simulink model "ToySystem"  (R2019b)
settings: Solver=VariableStepAuto  StartTime=0.0  StopTime=10.0  RelTol=1e-3
undefined symbols (not defined in the file or in its folder): b1, b2, Cp_wall, D, dH, dH1, dH2, f, f1, f2, Fluid, Fluid1, Fluid2, H, HTC, HTC1, HTC2, HTC_method, HTC_method1, HTC_method2, KL, KL1, KL2, L, L1, L2, M_wall, Nu_lam1, Nu_lam2, P_init, PAF, Pamb, Pass1, Pass2, rev_comms_sink, Tw_init, v, W1, W2
libraries: DAEMOT_Lib x21
(part 2 of 2)

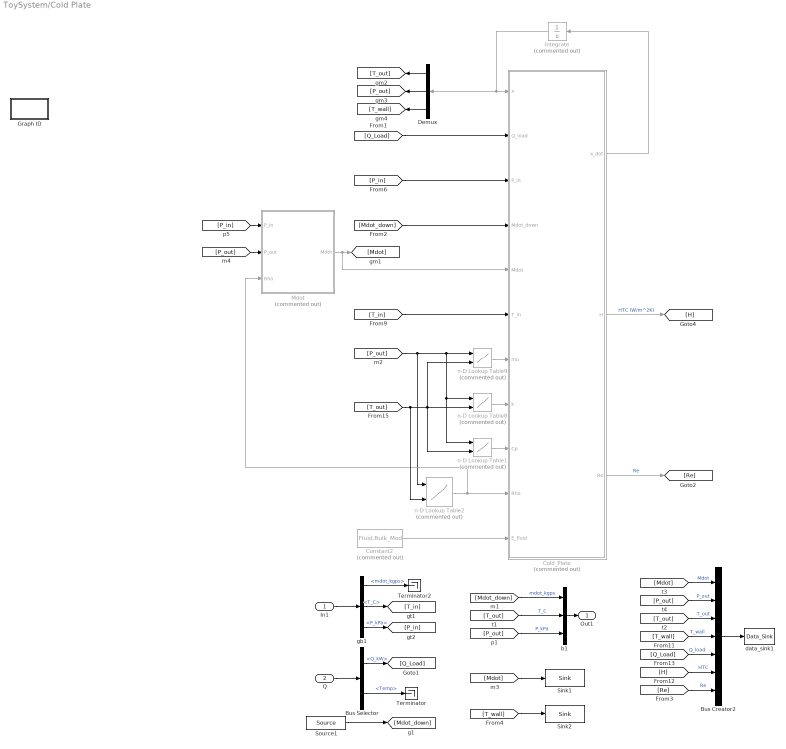
== system ToySystem/Cold Plate ==
  In1 : Inport
  Q : Inport  Port=2
  Bus Creator2 : BusCreator  Inputs=7
  Bus Selector : BusSelector  OutputSignals=Q_kW,Temp
  Cold_Plate : MATLAB Function  Commented=on  TreatAsAtomicUnit=on
  Constant2 : Constant  Commented=on  Value=Fluid.Bulk_Mod
  Demux : Demux  Outputs=3
  Graph ID : Subsystem  mask(Automated Graph Identifier){skip=off, graphType=HeatLoad, downCompType=SplitJunction, downCompPath=ToySystem/Junction, upCompType=Tank,Source, upCompPath=ToySystem/Tank 1,ToySystem/Generic Source1, spec=0}
      mask prompts: skip "Skip this block?"; graphType "Graph Type"; downCompType "Downstream Component Type"; downCompPath "Downstream Component Path"; upCompType "Upstream Component Type"; upCompPath "Upstream Component Path"; spec "Special"
      mask help: This block is used to generate directed graphs from DAEMOT models.
      mask init:
      | graph_connections()
      mask TypeOptions graphType: Tank | HeatExchanger | HeatLoad | SplitJunction | Source | Sink
      mask Callback graphType:
      | % grab the Simulink Mask object for this block
      | maskObj = Simulink.Mask.get(gcb);
      | 
      | % assign the popup with a list of graph options
      | maskObj.Parameters(2).TypeOptions = generateGraphList();
  Integrate : Integrator  Commented=on  InitialCondition=[T_init P_init Tw_init]
  Mdot : MATLAB Function  Commented=on  TreatAsAtomicUnit=on
  Sink1 : DAEMOT_Lib/Support Functions/Sink
      settings: SourceProductName=DAEMOT Toolset
  Sink2 : DAEMOT_Lib/Support Functions/Sink
      settings: SourceProductName=DAEMOT Toolset
  Source1 : DAEMOT_Lib/Support Functions/Source
      settings: SourceProductName=DAEMOT Toolset
  Terminator : Terminator
  Terminator2 : Terminator
  b1 : BusCreator  Inputs=3
  data_sink1 : DAEMOT_Lib/Support Functions/Data_Sink
      settings: SourceProductName=DAEMOT Toolset
  gb1 : BusSelector  OutputSignals=mdot_kgps,T_C,P_kPa
  n-D Lookup Table1 : Lookup_n-D  Commented=on  BreakpointsForDimension1=Fluid.P  BreakpointsForDimension2=Fluid.T  BreakpointsForDimension3=[5, 7]  Table=Fluid.C_pt  ExtrapMethod=Clip  UseLastTableValue=on  RndMeth=Simplest  InputSameDT=on
  n-D Lookup Table2 : Lookup_n-D  Commented=on  BreakpointsForDimension1=Fluid.P  BreakpointsForDimension2=Fluid.T  BreakpointsForDimension3=[5, 7]  Table=Fluid.Rho_pt  ExtrapMethod=Clip  UseLastTableValue=on  RndMeth=Simplest  InputSameDT=on
  n-D Lookup Table8 : Lookup_n-D  Commented=on  BreakpointsForDimension1=Fluid.P  BreakpointsForDimension2=Fluid.T  BreakpointsForDimension3=[5, 7]  Table=Fluid.K_pt  ExtrapMethod=Clip  UseLastTableValue=on  RndMeth=Simplest  InputSameDT=on
  n-D Lookup Table9 : Lookup_n-D  Commented=on  BreakpointsForDimension1=Fluid.P  BreakpointsForDimension2=Fluid.T  BreakpointsForDimension3=[5, 7]  Table=Fluid.Mu_pt  ExtrapMethod=Clip  UseLastTableValue=on  RndMeth=Simplest  InputSameDT=on
  Out1 : Outport  VectorParamsAs1DForOutWhenUnconnected=off
  wires:
  Bus Selector/2 -> Terminator/1  "<Temp>"
  [T_wall] -> Sink2/1
  Bus Selector/1 -> [Q_Load]  "<Q_kW>"
  Q/1 -> Bus Selector/1
  [Re] -> Bus Creator2/7  "Re"
  Cold_Plate/3(Re) -> [Re]  "Re"
  [P_out] -> n-D Lookup Table9/1, n-D Lookup Table8/1, n-D Lookup Table1/1, n-D Lookup Table2/1
  Demux/3 -> [T_wall]
  Demux/1 -> [T_out]
  Demux/2 -> [P_out]
  [P_out] -> Mdot/2(P_out)
  [P_in] -> Mdot/1(P_in)
  Mdot/1(Mdot) -> Cold_Plate/5(Mdot), [Mdot]
  n-D Lookup Table2/1 -> Cold_Plate/10(Rho), Mdot/3(Rho)
  [P_in] -> Cold_Plate/3(P_in)
  [Mdot_down] -> Cold_Plate/4(Mdot_down)
  Constant2/1 -> Cold_Plate/11(E_fluid)
  n-D Lookup Table1/1 -> Cold_Plate/9(Cp)
  Integrate/1 -> Demux/1, Cold_Plate/1(x)
  [T_out] -> n-D Lookup Table8/2, n-D Lookup Table1/2, n-D Lookup Table9/2, n-D Lookup Table2/2
  n-D Lookup Table9/1 -> Cold_Plate/7(mu)
  n-D Lookup Table8/1 -> Cold_Plate/8(k)
  [H] -> Bus Creator2/6  "HTC"
  Cold_Plate/2(H) -> [H]  "HTC (W/m^2K)"
  [Mdot] -> Bus Creator2/1  "Mdot"
  [Q_Load] -> Bus Creator2/5  "Q_load"
  [P_out] -> Bus Creator2/2  "P_out"
  [T_out] -> Bus Creator2/3  "T_out"
  [T_wall] -> Bus Creator2/4  "T_wall"
  Bus Creator2/1 -> data_sink1/1
  Cold_Plate/1(x_dot) -> Integrate/1
  [T_in] -> Cold_Plate/6(T_in)
  Source1/1 -> [Mdot_down]
  [Q_Load] -> Cold_Plate/2(Q_load)
  [Mdot] -> Sink1/1
  gb1/3 -> [P_in]  "<P_kPa>"
  [P_out] -> b1/3  "P_kPa"
  In1/1 -> gb1/1
  gb1/1 -> Terminator2/1  "<mdot_kgps>"
  [T_out] -> b1/2  "T_C"
  gb1/2 -> [T_in]  "<T_C>"
  [Mdot_down] -> b1/1  "mdot_kgps"
  b1/1 -> Out1/1

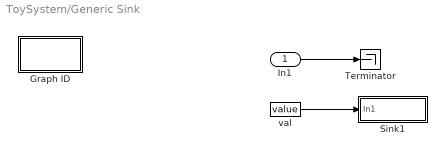
== system ToySystem/Generic Sink ==
  In1 : Inport
  Graph ID : Subsystem  mask(Automated Graph Identifier){skip=off, graphType=Sink, downCompType=, downCompPath=, upCompType=HeatExchanger, upCompPath=ToySystem/HX, spec=0}
      mask prompts: skip "Skip this block?"; graphType "Graph Type"; downCompType "Downstream Component Type"; downCompPath "Downstream Component Path"; upCompType "Upstream Component Type"; upCompPath "Upstream Component Path"; spec "Special"
      mask help: This block is used to generate directed graphs from DAEMOT models.
      mask init:
      | graph_connections()
      mask TypeOptions graphType: Tank | HeatExchanger | HeatLoad | SplitJunction | Source | Sink
      mask Callback graphType:
      | % grab the Simulink Mask object for this block
      | maskObj = Simulink.Mask.get(gcb);
      | 
      | % assign the popup with a list of graph options
      | maskObj.Parameters(2).TypeOptions = generateGraphList();
  Sink1 : Subsystem  LoadFcn=rev_comms_sink();  InitFcn=rev_comms_sink();  mask(Sink){}
      mask help: Used for sending data to the upstream component.
      settings: CopyFcn=rev_comms_sink();  NameChangeFcn=rev_comms_sink();
      mask Display: text(0.25,0.5,'Sink')
  Terminator : Terminator
  val : Constant  Value=value
  wires:
  val/1 -> Sink1/1(In1)
  In1/1 -> Terminator/1

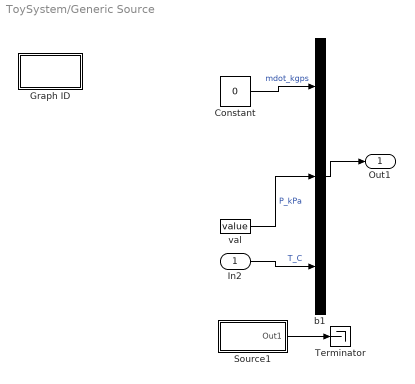
== system ToySystem/Generic Source ==
  In2 : Inport
  Constant : Constant  Value=0
  Graph ID : Subsystem  mask(Automated Graph Identifier){skip=off, graphType=Source, downCompType=HeatExchanger, downCompPath=ToySystem/HX, upCompType=, upCompPath=, spec=0}
      mask prompts: skip "Skip this block?"; graphType "Graph Type"; downCompType "Downstream Component Type"; downCompPath "Downstream Component Path"; upCompType "Upstream Component Type"; upCompPath "Upstream Component Path"; spec "Special"
      mask help: This block is used to generate directed graphs from DAEMOT models.
      mask init:
      | graph_connections()
      mask TypeOptions graphType: Tank | HeatExchanger | HeatLoad | SplitJunction | Source | Sink
      mask Callback graphType:
      | % grab the Simulink Mask object for this block
      | maskObj = Simulink.Mask.get(gcb);
      | 
      | % assign the popup with a list of graph options
      | maskObj.Parameters(2).TypeOptions = generateGraphList();
  Source1 : Subsystem  mask(Source){}
      mask help: Used for receiving data from the downstream component.
      mask init:
      | n_src = gcb;
      | n_src = str2num(n_src(end));
      | try
      |     rev_comms_source(n_src);
      | catch
      | 
      | end
      mask Display: text(0.25,0.5,'Source')
  Terminator : Terminator
  b1 : BusCreator  Inputs=3
  val : Constant  Value=value
  Out1 : Outport  VectorParamsAs1DForOutWhenUnconnected=off
  wires:
  val/1 -> b1/2  "P_kPa"
  b1/1 -> Out1/1
  Source1/1(Out1) -> Terminator/1
  Constant/1 -> b1/1  "mdot_kgps"
  In2/1 -> b1/3  "T_C"

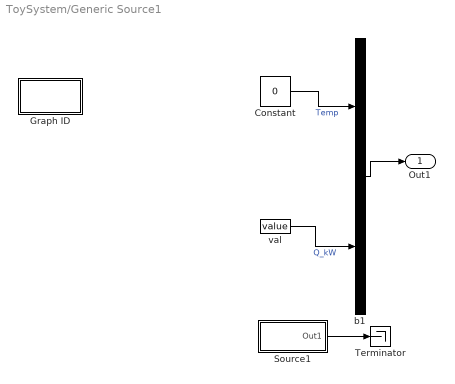
== system ToySystem/Generic Source1 ==
  Constant : Constant  Value=0
  Graph ID : Subsystem  mask(Automated Graph Identifier){skip=off, graphType=Source, downCompType=HeatLoad, downCompPath=ToySystem/Cold Plate, upCompType=, upCompPath=, spec=0}
      mask prompts: skip "Skip this block?"; graphType "Graph Type"; downCompType "Downstream Component Type"; downCompPath "Downstream Component Path"; upCompType "Upstream Component Type"; upCompPath "Upstream Component Path"; spec "Special"
      mask help: This block is used to generate directed graphs from DAEMOT models.
      mask init:
      | graph_connections()
      mask TypeOptions graphType: Tank | HeatExchanger | HeatLoad | SplitJunction | Source | Sink
      mask Callback graphType:
      | % grab the Simulink Mask object for this block
      | maskObj = Simulink.Mask.get(gcb);
      | 
      | % assign the popup with a list of graph options
      | maskObj.Parameters(2).TypeOptions = generateGraphList();
  Source1 : Subsystem  mask(Source){}
      mask help: Used for receiving data from the downstream component.
      mask init:
      | n_src = gcb;
      | n_src = str2num(n_src(end));
      | try
      |     rev_comms_source(n_src);
      | catch
      | 
      | end
      mask Display: text(0.25,0.5,'Source')
  Terminator : Terminator
  b1 : BusCreator  Inputs=2
  val : Constant  Value=value
  Out1 : Outport  VectorParamsAs1DForOutWhenUnconnected=off
  wires:
  Constant/1 -> b1/1  "Temp"
  Source1/1(Out1) -> Terminator/1
  b1/1 -> Out1/1
  val/1 -> b1/2  "Q_kW"

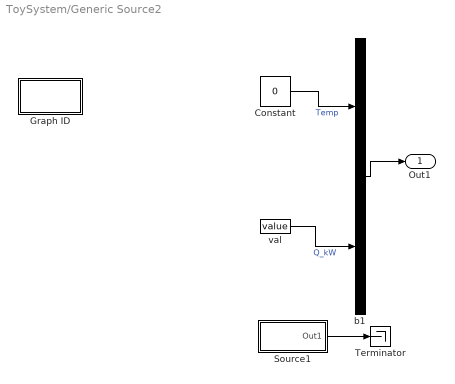
== system ToySystem/Generic Source2 ==
  Constant : Constant  Value=0
  Graph ID : Subsystem  mask(Automated Graph Identifier){skip=off, graphType=Source, downCompType=Tank, downCompPath=ToySystem/Tank 1, upCompType=, upCompPath=, spec=0}
      mask prompts: skip "Skip this block?"; graphType "Graph Type"; downCompType "Downstream Component Type"; downCompPath "Downstream Component Path"; upCompType "Upstream Component Type"; upCompPath "Upstream Component Path"; spec "Special"
      mask help: This block is used to generate directed graphs from DAEMOT models.
      mask init:
      | graph_connections()
      mask TypeOptions graphType: Tank | HeatExchanger | HeatLoad | SplitJunction | Source | Sink
      mask Callback graphType:
      | % grab the Simulink Mask object for this block
      | maskObj = Simulink.Mask.get(gcb);
      | 
      | % assign the popup with a list of graph options
      | maskObj.Parameters(2).TypeOptions = generateGraphList();
  Source1 : Subsystem  mask(Source){}
      mask help: Used for receiving data from the downstream component.
      mask init:
      | n_src = gcb;
      | n_src = str2num(n_src(end));
      | try
      |     rev_comms_source(n_src);
      | catch
      | 
      | end
      mask Display: text(0.25,0.5,'Source')
  Terminator : Terminator
  b1 : BusCreator  Inputs=2
  val : Constant  Value=value
  Out1 : Outport  VectorParamsAs1DForOutWhenUnconnected=off
  wires:
  val/1 -> b1/2  "Q_kW"
  b1/1 -> Out1/1
  Source1/1(Out1) -> Terminator/1
  Constant/1 -> b1/1  "Temp"

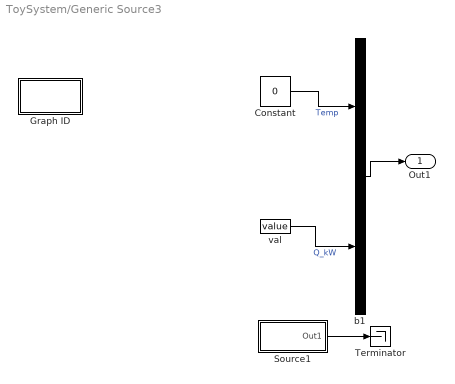
== system ToySystem/Generic Source3 ==
  Constant : Constant  Value=0
  Graph ID : Subsystem  mask(Automated Graph Identifier){skip=off, graphType=Source, downCompType=Tank, downCompPath=ToySystem/Tank 2, upCompType=, upCompPath=, spec=0}
      mask prompts: skip "Skip this block?"; graphType "Graph Type"; downCompType "Downstream Component Type"; downCompPath "Downstream Component Path"; upCompType "Upstream Component Type"; upCompPath "Upstream Component Path"; spec "Special"
      mask help: This block is used to generate directed graphs from DAEMOT models.
      mask init:
      | graph_connections()
      mask TypeOptions graphType: Tank | HeatExchanger | HeatLoad | SplitJunction | Source | Sink
      mask Callback graphType:
      | % grab the Simulink Mask object for this block
      | maskObj = Simulink.Mask.get(gcb);
      | 
      | % assign the popup with a list of graph options
      | maskObj.Parameters(2).TypeOptions = generateGraphList();
  Source1 : Subsystem  mask(Source){}
      mask help: Used for receiving data from the downstream component.
      mask init:
      | n_src = gcb;
      | n_src = str2num(n_src(end));
      | try
      |     rev_comms_source(n_src);
      | catch
      | 
      | end
      mask Display: text(0.25,0.5,'Source')
  Terminator : Terminator
  b1 : BusCreator  Inputs=2
  val : Constant  Value=value
  Out1 : Outport  VectorParamsAs1DForOutWhenUnconnected=off
  wires:
  Constant/1 -> b1/1  "Temp"
  Source1/1(Out1) -> Terminator/1
  b1/1 -> Out1/1
  val/1 -> b1/2  "Q_kW"

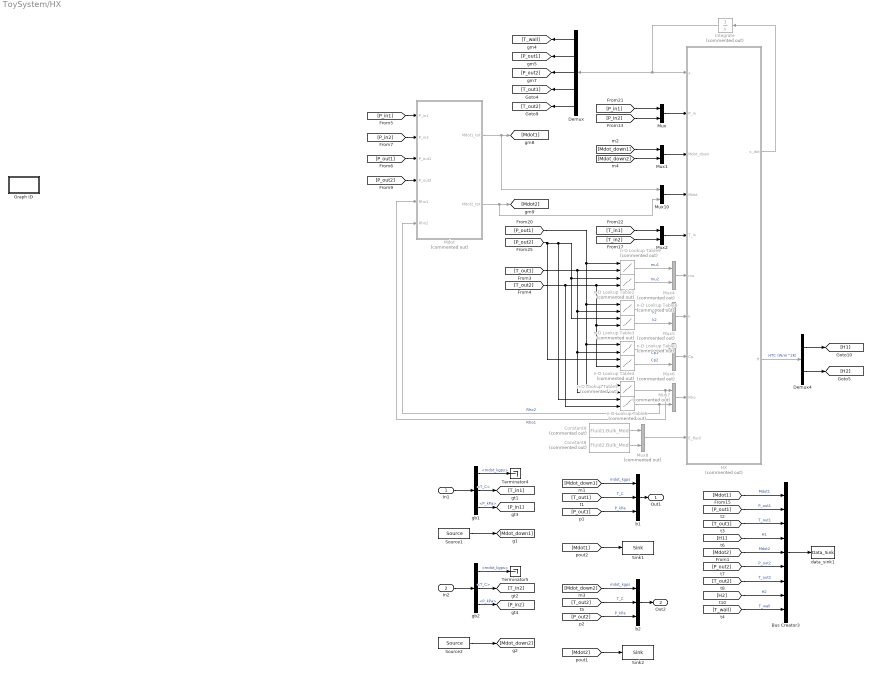
== system ToySystem/HX ==
  In1 : Inport
  In2 : Inport  Port=2
  Bus Creator3 : BusCreator  Inputs=9
  Constant8 : Constant  Commented=on  Value=Fluid2.Bulk_Mod
  Constant9 : Constant  Commented=on  Value=Fluid1.Bulk_Mod
  Demux : Demux  Outputs=5
  Demux4 : Demux  Outputs=2
  Graph ID : Subsystem  mask(Automated Graph Identifier){skip=off, graphType=HeatExchanger, downCompType=Sink,SplitJunction, downCompPath=ToySystem/Generic Sink,ToySystem/Junction1, upCompType=Source,SplitJunction, upCompPath=ToySystem/Generic Source,ToySystem/Junction, spec=0}
      mask prompts: skip "Skip this block?"; graphType "Graph Type"; downCompType "Downstream Component Type"; downCompPath "Downstream Component Path"; upCompType "Upstream Component Type"; upCompPath "Upstream Component Path"; spec "Special"
      mask help: This block is used to generate directed graphs from DAEMOT models.
      mask init:
      | graph_connections()
      mask TypeOptions graphType: Tank | HeatExchanger | HeatLoad | SplitJunction | Source | Sink
      mask Callback graphType:
      | % grab the Simulink Mask object for this block
      | maskObj = Simulink.Mask.get(gcb);
      | 
      | % assign the popup with a list of graph options
      | maskObj.Parameters(2).TypeOptions = generateGraphList();
  HX : MATLAB Function  Commented=on  TreatAsAtomicUnit=on
  Integrate : Integrator  Commented=on  InitialCondition=[Tw_init P1_init P2_init T1_init T2_init]
  Mdot : MATLAB Function  Commented=on  TreatAsAtomicUnit=on
  Mux{,1..2,10} (4 alike) : Mux  Inputs=2
  Mux{4..8} (5 alike) : Mux  Commented=on  Inputs=2
  Sink1 : DAEMOT_Lib/Support Functions/Sink
      settings: SourceProductName=DAEMOT Toolset
  Sink2 : DAEMOT_Lib/Support Functions/Sink
      settings: SourceProductName=DAEMOT Toolset
  Source1 : DAEMOT_Lib/Support Functions/Source
      settings: SourceProductName=DAEMOT Toolset
  Source2 : DAEMOT_Lib/Support Functions/Source
      settings: SourceProductName=DAEMOT Toolset
  Terminator4 : Terminator
  Terminator5 : Terminator
  b1 : BusCreator  Inputs=3
  b2 : BusCreator  Inputs=3
  data_sink1 : DAEMOT_Lib/Support Functions/Data_Sink
      settings: SourceProductName=DAEMOT Toolset
  gb1 : BusSelector  OutputSignals=mdot_kgps,T_C,P_kPa
  gb2 : BusSelector  OutputSignals=mdot_kgps,T_C,P_kPa
  n-D Lookup Table1 : Lookup_n-D  Commented=on  BreakpointsForDimension1=Fluid1.P  BreakpointsForDimension2=Fluid1.T  BreakpointsForDimension3=[5, 7]  Table=Fluid1.C_pt  ExtrapMethod=Clip  RndMeth=Simplest  InputSameDT=on
  n-D Lookup Table2 : Lookup_n-D  Commented=on  BreakpointsForDimension1=Fluid2.P  BreakpointsForDimension2=Fluid2.T  BreakpointsForDimension3=[5, 7]  Table=Fluid2.Mu_pt  ExtrapMethod=Clip  UseLastTableValue=on  RndMeth=Simplest  InputSameDT=on
  n-D Lookup Table3 : Lookup_n-D  Commented=on  BreakpointsForDimension1=Fluid2.P  BreakpointsForDimension2=Fluid2.T  BreakpointsForDimension3=[5, 7]  Table=Fluid2.K_pt  ExtrapMethod=Clip  UseLastTableValue=on  RndMeth=Simplest  InputSameDT=on
  n-D Lookup Table4 : Lookup_n-D  Commented=on  BreakpointsForDimension1=Fluid2.P  BreakpointsForDimension2=Fluid2.T  BreakpointsForDimension3=[5, 7]  Table=Fluid2.C_pt  ExtrapMethod=Clip  UseLastTableValue=on  RndMeth=Simplest  InputSameDT=on
  n-D Lookup Table5 : Lookup_n-D  Commented=on  BreakpointsForDimension1=Fluid1.P  BreakpointsForDimension2=Fluid1.T  BreakpointsForDimension3=[5, 7]  Table=Fluid1.Rho_pt  ExtrapMethod=Clip  UseLastTableValue=on  RndMeth=Simplest  InputSameDT=on
  n-D Lookup Table6 : Lookup_n-D  Commented=on  BreakpointsForDimension1=Fluid2.P  BreakpointsForDimension2=Fluid2.T  BreakpointsForDimension3=[5, 7]  Table=Fluid2.Rho_pt  ExtrapMethod=Clip  UseLastTableValue=on  RndMeth=Simplest  InputSameDT=on
  n-D Lookup Table8 : Lookup_n-D  Commented=on  BreakpointsForDimension1=Fluid1.P  BreakpointsForDimension2=Fluid1.T  BreakpointsForDimension3=[5, 7]  Table=Fluid1.K_pt  ExtrapMethod=Clip  UseLastTableValue=on  RndMeth=Simplest  InputSameDT=on
  n-D Lookup Table9 : Lookup_n-D  Commented=on  BreakpointsForDimension1=Fluid1.P  BreakpointsForDimension2=Fluid1.T  BreakpointsForDimension3=[5, 7]  Table=Fluid1.Mu_pt  ExtrapMethod=Clip  UseLastTableValue=on  RndMeth=Simplest  InputSameDT=on
  Out1 : Outport  VectorParamsAs1DForOutWhenUnconnected=off
  Out2 : Outport  Port=2  VectorParamsAs1DForOutWhenUnconnected=off
  wires:
  [P_out1] -> Mdot/3(P_out1)
  Mdot/2(Mdot2_tot) -> [Mdot2], Mux10/2
  Mux10/1 -> HX/4(Mdot)
  Mdot/1(Mdot1_tot) -> [Mdot1], Mux10/1
  Demux/5 -> [T_out2]
  Demux/4 -> [T_out1]
  [P_out2] -> Mdot/4(P_out2)
  [P_in2] -> Mdot/2(P_in2)
  n-D Lookup Table6/1 -> Mux7/2, Mdot/6(Rho2)  "Rho2"
  [P_in1] -> Mdot/1(P_in1)
  Bus Creator3/1 -> data_sink1/1
  [Mdot1] -> Bus Creator3/1  "Mdot1"
  [P_out1] -> Bus Creator3/2  "P_out1"
  [T_wall] -> Bus Creator3/9  "T_wall"
  [T_out1] -> Bus Creator3/3  "T_out1"
  [H1] -> Bus Creator3/4  "H1"
  [Mdot2] -> Bus Creator3/5  "Mdot2"
  [P_out2] -> Bus Creator3/6  "P_out2"
  [T_out2] -> Bus Creator3/7  "T_out2"
  [H2] -> Bus Creator3/8  "H2"
  Constant8/1 -> Mux8/2
  Constant9/1 -> Mux8/1
  Demux/3 -> [P_out2]
  Demux4/2 -> [H2]
  Demux4/1 -> [H1]
  Mux8/1 -> HX/10(E_fluid)
  Mux7/1 -> HX/9(Rho)
  n-D Lookup Table4/1 -> Mux6/2  "Cp2"
  Mux6/1 -> HX/8(Cp)
  n-D Lookup Table3/1 -> Mux5/2  "k2"
  Mux5/1 -> HX/7(k)
  [T_out2] -> n-D Lookup Table6/2, n-D Lookup Table2/2, n-D Lookup Table4/2, n-D Lookup Table3/2
  [P_out2] -> n-D Lookup Table2/1, n-D Lookup Table3/1, n-D Lookup Table6/1, n-D Lookup Table4/1
  n-D Lookup Table2/1 -> Mux4/2  "mu2"
  Mux4/1 -> HX/6(mu)
  [T_in2] -> Mux2/2
  Mux2/1 -> HX/5(T_in)
  [Mdot_down2] -> Mux1/2
  Mux1/1 -> HX/3(Mdot_down)
  [P_in2] -> Mux/2
  Mux/1 -> HX/2(P_in)
  [Mdot2] -> Sink2/1
  [P_out2] -> b2/3  "P_kPa"
  [T_out2] -> b2/2  "T_C"
  [Mdot_down2] -> b2/1  "mdot_kgps"
  b2/1 -> Out2/1
  Source2/1 -> [Mdot_down2]
  gb2/3 -> [P_in2]  "<P_kPa>"
  In2/1 -> gb2/1
  gb2/1 -> Terminator5/1  "<mdot_kgps>"
  gb2/2 -> [T_in2]  "<T_C>"
  n-D Lookup Table5/1 -> Mux7/1, Mdot/5(Rho1)  "Rho1"
  n-D Lookup Table1/1 -> Mux6/1  "Cp1"
  [P_out1] -> n-D Lookup Table9/1, n-D Lookup Table8/1, n-D Lookup Table1/1, n-D Lookup Table5/1
  [T_out1] -> n-D Lookup Table8/2, n-D Lookup Table1/2, n-D Lookup Table5/2, n-D Lookup Table9/2
  n-D Lookup Table9/1 -> Mux4/1  "mu1"
  n-D Lookup Table8/1 -> Mux5/1  "k1"
  HX/2(H) -> Demux4/1  "HTC (W/m^2K)"
  Demux/2 -> [P_out1]
  Demux/1 -> [T_wall]
  Integrate/1 -> HX/1(x), Demux/1
  HX/1(x_dot) -> Integrate/1
  [T_in1] -> Mux2/1
  [Mdot_down1] -> Mux1/1
  Source1/1 -> [Mdot_down1]
  [P_in1] -> Mux/1
  [Mdot1] -> Sink1/1
  gb1/3 -> [P_in1]  "<P_kPa>"
  [P_out1] -> b1/3  "P_kPa"
  In1/1 -> gb1/1
  gb1/1 -> Terminator4/1  "<mdot_kgps>"
  [T_out1] -> b1/2  "T_C"
  gb1/2 -> [T_in1]  "<T_C>"
  [Mdot_down1] -> b1/1  "mdot_kgps"
  b1/1 -> Out1/1

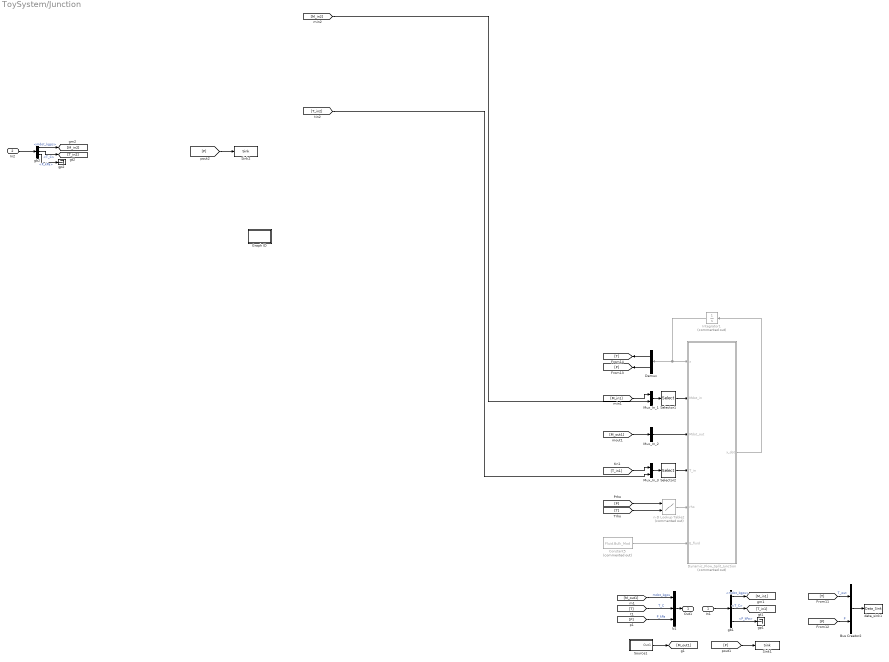
== system ToySystem/Junction ==
  In1 : Inport
  In2 : Inport  Port=2
  Bus Creator2 : BusCreator  Inputs=2
  Constant5 : Constant  Commented=on  Value=Fluid.Bulk_Mod
  Demux : Demux  Outputs=2
  Dynamic_Flow_Split_Junction : MATLAB Function  Commented=on  TreatAsAtomicUnit=on
  Graph ID : Subsystem  mask(Automated Graph Identifier){skip=off, graphType=SplitJunction, downCompType=HeatExchanger, downCompPath=ToySystem/HX, upCompType=HeatLoad,Tank, upCompPath=ToySystem/Cold Plate,ToySystem/Tank 2, spec=0}
      mask prompts: skip "Skip this block?"; graphType "Graph Type"; downCompType "Downstream Component Type"; downCompPath "Downstream Component Path"; upCompType "Upstream Component Type"; upCompPath "Upstream Component Path"; spec "Special"
      mask help: This block is used to generate directed graphs from DAEMOT models.
      mask init:
      | graph_connections()
      mask TypeOptions graphType: Tank | HeatExchanger | HeatLoad | SplitJunction | Source | Sink
      mask Callback graphType:
      | % grab the Simulink Mask object for this block
      | maskObj = Simulink.Mask.get(gcb);
      | 
      | % assign the popup with a list of graph options
      | maskObj.Parameters(2).TypeOptions = generateGraphList();
  Integrator1 : Integrator  Commented=on  InitialCondition=[T_init P_init]
  Mux_In_1 : Mux  Inputs=2
  Mux_In_2 : Mux  Inputs=1
  Mux_In_3 : Mux  Inputs=2
  Selector1 : Selector  InputPortWidth=2  IndexOptions=Index vector (dialog)  Indices=[1 2 ]  OutputSizes=1
  Selector2 : Selector  InputPortWidth=2  IndexOptions=Index vector (dialog)  Indices=[1 2 ]  OutputSizes=1
  Sink1 : DAEMOT_Lib/Support Functions/Sink
      settings: SourceProductName=DAEMOT Toolset
  Sink2 : DAEMOT_Lib/Support Functions/Sink
      settings: SourceProductName=DAEMOT Toolset
  Source1 : Subsystem
      mask init:
      | n_src = gcb;
      | n_src = str2num(n_src(end));
      | 
      | rev_comms_source(n_src);
      mask Display: text(0.25,0.5,'Source')
  b1 : BusCreator  Inputs=3
  data_sink1 : DAEMOT_Lib/Support Functions/Data_Sink
      settings: SourceProductName=DAEMOT Toolset
  gb1 : BusSelector  OutputSignals=mdot_kgps,T_C,P_kPa
  gb2 : BusSelector  OutputSignals=mdot_kgps,T_C,P_kPa
  gp1 : Terminator
  gp2 : Terminator
  n-D Lookup Table2 : Lookup_n-D  Commented=on  BreakpointsForDimension1=Fluid.P  BreakpointsForDimension2=Fluid.T  BreakpointsForDimension3=[5, 7]  Table=Fluid.Rho_pt  ExtrapMethod=Clip  UseLastTableValue=on  RndMeth=Simplest  InputSameDT=on
  Out1 : Outport  VectorParamsAs1DForOutWhenUnconnected=off
  wires:
  Selector2/1 -> Dynamic_Flow_Split_Junction/4(T_in)
  Demux/2 -> [P]
  Demux/1 -> [T]
  [T] -> n-D Lookup Table2/2
  [P] -> n-D Lookup Table2/1
  n-D Lookup Table2/1 -> Dynamic_Flow_Split_Junction/5(rho)
  Constant5/1 -> Dynamic_Flow_Split_Junction/6(E_fluid)
  Selector1/1 -> Dynamic_Flow_Split_Junction/2(Mdot_in)
  Integrator1/1 -> Dynamic_Flow_Split_Junction/1(x), Demux/1
  [P] -> Bus Creator2/2  "P"
  [T] -> Bus Creator2/1  "T_out"
  Bus Creator2/1 -> data_sink1/1
  Dynamic_Flow_Split_Junction/1(x_dot) -> Integrator1/1
  [P] -> Sink1/1
  [T_in1] -> Mux_In_3/1
  [M_out1] -> Mux_In_2/1
  [M_in1] -> Mux_In_1/1
  Mux_In_2/1 -> Dynamic_Flow_Split_Junction/3(Mdot_out)
  Mux_In_1/1 -> Selector1/1
  Mux_In_3/1 -> Selector2/1
  gb1/3 -> gp1/1  "<P_kPa>"
  [P] -> b1/3  "P_kPa"
  In1/1 -> gb1/1
  Source1/1(Out1) -> [M_out1]
  gb1/1 -> [M_in1]  "<mdot_kgps>"
  [T] -> b1/2  "T_C"
  gb1/2 -> [T_in1]  "<T_C>"
  [M_out1] -> b1/1  "mdot_kgps"
  b1/1 -> Out1/1
  In2/1 -> gb2/1
  gb2/1 -> [M_in2]  "<mdot_kgps>"
  gb2/2 -> [T_in2]  "<T_C>"
  gb2/3 -> gp2/1  "<P_kPa>"
  [P] -> Sink2/1
  [M_in2] -> Mux_In_1/2
  [T_in2] -> Mux_In_3/2

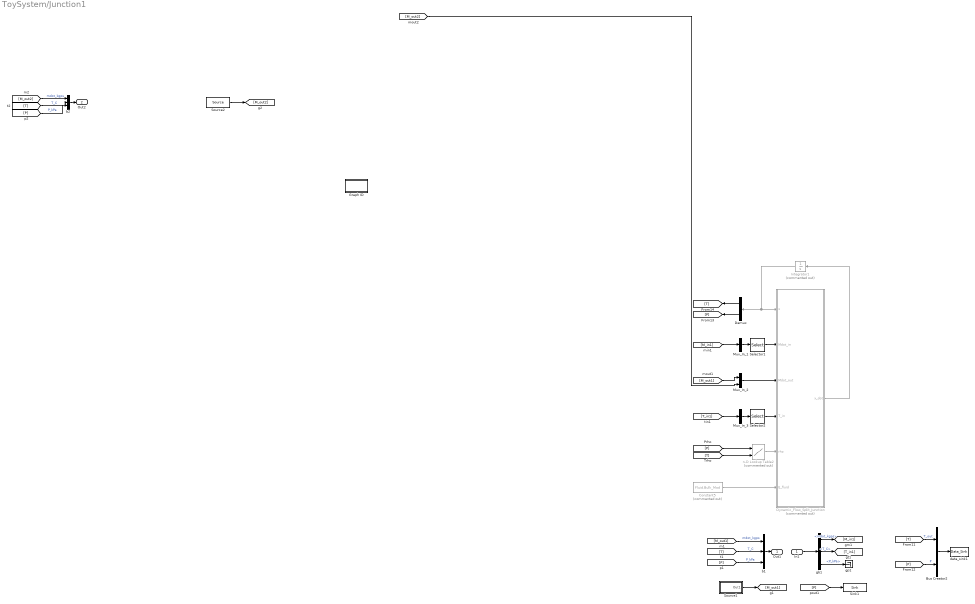
== system ToySystem/Junction1 ==
  In1 : Inport
  Bus Creator2 : BusCreator  Inputs=2
  Constant5 : Constant  Commented=on  Value=Fluid.Bulk_Mod
  Demux : Demux  Outputs=2
  Dynamic_Flow_Split_Junction : MATLAB Function  Commented=on  TreatAsAtomicUnit=on
  Graph ID : Subsystem  mask(Automated Graph Identifier){skip=off, graphType=SplitJunction, downCompType=Tank,Tank, downCompPath=ToySystem/Tank 1,ToySystem/Tank 2, upCompType=HeatExchanger, upCompPath=ToySystem/HX, spec=0}
      mask prompts: skip "Skip this block?"; graphType "Graph Type"; downCompType "Downstream Component Type"; downCompPath "Downstream Component Path"; upCompType "Upstream Component Type"; upCompPath "Upstream Component Path"; spec "Special"
      mask help: This block is used to generate directed graphs from DAEMOT models.
      mask init:
      | graph_connections()
      mask TypeOptions graphType: Tank | HeatExchanger | HeatLoad | SplitJunction | Source | Sink
      mask Callback graphType:
      | % grab the Simulink Mask object for this block
      | maskObj = Simulink.Mask.get(gcb);
      | 
      | % assign the popup with a list of graph options
      | maskObj.Parameters(2).TypeOptions = generateGraphList();
  Integrator1 : Integrator  Commented=on  InitialCondition=[T_init P_init]
  Mux_In_1 : Mux  Inputs=1
  Mux_In_2 : Mux  Inputs=2
  Mux_In_3 : Mux  Inputs=1
  Selector1 : Selector  InputPortWidth=1  IndexOptions=Index vector (dialog)  Indices=[1 ]  OutputSizes=1
  Selector2 : Selector  InputPortWidth=1  IndexOptions=Index vector (dialog)  Indices=[1 ]  OutputSizes=1
  Sink1 : DAEMOT_Lib/Support Functions/Sink
      settings: SourceProductName=DAEMOT Toolset
  Source1 : Subsystem
      mask init:
      | n_src = gcb;
      | n_src = str2num(n_src(end));
      | 
      | rev_comms_source(n_src);
      mask Display: text(0.25,0.5,'Source')
  Source2 : DAEMOT_Lib/Support Functions/Source
      settings: SourceProductName=DAEMOT Toolset
  b1 : BusCreator  Inputs=3
  b2 : BusCreator  Inputs=3
  data_sink1 : DAEMOT_Lib/Support Functions/Data_Sink
      settings: SourceProductName=DAEMOT Toolset
  gb1 : BusSelector  OutputSignals=mdot_kgps,T_C,P_kPa
  gp1 : Terminator
  n-D Lookup Table2 : Lookup_n-D  Commented=on  BreakpointsForDimension1=Fluid.P  BreakpointsForDimension2=Fluid.T  BreakpointsForDimension3=[5, 7]  Table=Fluid.Rho_pt  ExtrapMethod=Clip  UseLastTableValue=on  RndMeth=Simplest  InputSameDT=on
  Out1 : Outport  VectorParamsAs1DForOutWhenUnconnected=off
  Out2 : Outport  Port=2
  wires:
  b1/1 -> Out1/1
  [M_out1] -> b1/1  "mdot_kgps"
  gb1/2 -> [T_in1]  "<T_C>"
  [T] -> b1/2  "T_C"
  gb1/1 -> [M_in1]  "<mdot_kgps>"
  Source1/1(Out1) -> [M_out1]
  In1/1 -> gb1/1
  [P] -> b1/3  "P_kPa"
  gb1/3 -> gp1/1  "<P_kPa>"
  Mux_In_3/1 -> Selector2/1
  Mux_In_1/1 -> Selector1/1
  Mux_In_2/1 -> Dynamic_Flow_Split_Junction/3(Mdot_out)
  [M_in1] -> Mux_In_1/1
  [M_out1] -> Mux_In_2/1
  [T_in1] -> Mux_In_3/1
  [P] -> Sink1/1
  Dynamic_Flow_Split_Junction/1(x_dot) -> Integrator1/1
  Bus Creator2/1 -> data_sink1/1
  [T] -> Bus Creator2/1  "T_out"
  [P] -> Bus Creator2/2  "P"
  Integrator1/1 -> Demux/1, Dynamic_Flow_Split_Junction/1(x)
  Selector1/1 -> Dynamic_Flow_Split_Junction/2(Mdot_in)
  Constant5/1 -> Dynamic_Flow_Split_Junction/6(E_fluid)
  n-D Lookup Table2/1 -> Dynamic_Flow_Split_Junction/5(rho)
  [P] -> n-D Lookup Table2/1
  [T] -> n-D Lookup Table2/2
  Demux/1 -> [T]
  Demux/2 -> [P]
  Selector2/1 -> Dynamic_Flow_Split_Junction/4(T_in)
  [M_out2] -> b2/1  "mdot_kgps"
  [T] -> b2/2  "T_C"
  [P] -> b2/3  "P_kPa"
  b2/1 -> Out2/1
  Source2/1 -> [M_out2]
  [M_out2] -> Mux_In_2/2

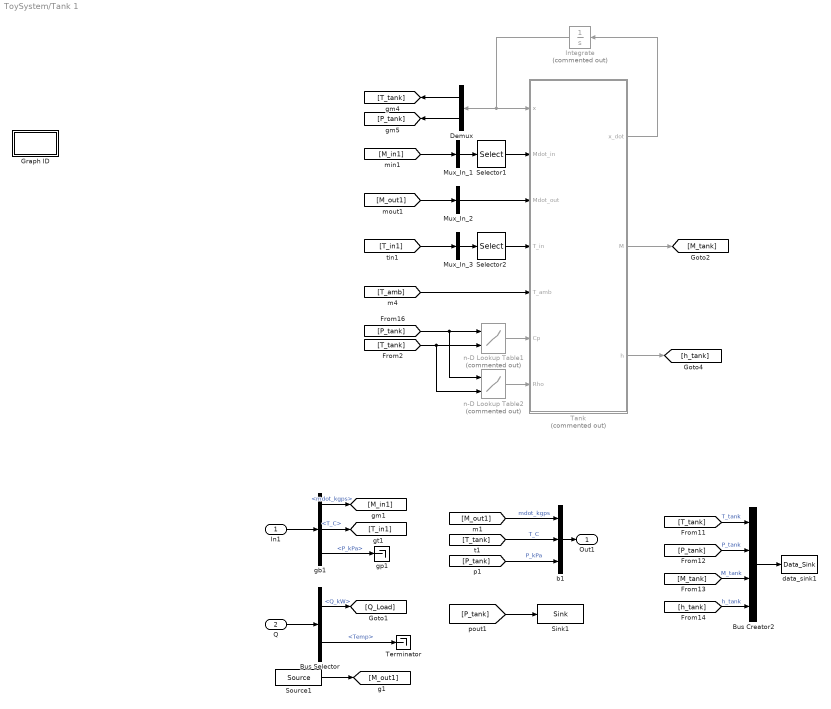
== system ToySystem/Tank 1 ==
  In1 : Inport
  Q : Inport  Port=2
  Bus Creator2 : BusCreator  Inputs=4
  Bus Selector : BusSelector  OutputSignals=Q_kW,Temp
  Demux : Demux  Outputs=2
  Graph ID : Subsystem  mask(Automated Graph Identifier){skip=off, graphType=Tank, downCompType=HeatLoad, downCompPath=ToySystem/Cold Plate, upCompType=SplitJunction,Source, upCompPath=ToySystem/Junction1,ToySystem/Generic Source2, spec=0}
      mask prompts: skip "Skip this block?"; graphType "Graph Type"; downCompType "Downstream Component Type"; downCompPath "Downstream Component Path"; upCompType "Upstream Component Type"; upCompPath "Upstream Component Path"; spec "Special"
      mask help: This block is used to generate directed graphs from DAEMOT models.
      mask init:
      | graph_connections()
      mask TypeOptions graphType: Tank | HeatExchanger | HeatLoad | SplitJunction | Source | Sink
      mask Callback graphType:
      | % grab the Simulink Mask object for this block
      | maskObj = Simulink.Mask.get(gcb);
      | 
      | % assign the popup with a list of graph options
      | maskObj.Parameters(2).TypeOptions = generateGraphList();
  Integrate : Integrator  Commented=on  InitialCondition=[T_init P_init]
  Mux_In_1 : Mux  Inputs=1
  Mux_In_2 : Mux  Inputs=1
  Mux_In_3 : Mux  Inputs=1
  Selector1 : Selector  InputPortWidth=1  IndexOptions=Index vector (dialog)  Indices=[1 ]  OutputSizes=1
  Selector2 : Selector  InputPortWidth=1  IndexOptions=Index vector (dialog)  Indices=[1 ]  OutputSizes=1
  Sink1 : DAEMOT_Lib/Support Functions/Sink
      settings: SourceProductName=DAEMOT Toolset
  Source1 : DAEMOT_Lib/Support Functions/Source
      settings: SourceProductName=DAEMOT Toolset
  Tank : MATLAB Function  Commented=on  TreatAsAtomicUnit=on
  Terminator : Terminator
  b1 : BusCreator  Inputs=3
  data_sink1 : DAEMOT_Lib/Support Functions/Data_Sink
      settings: SourceProductName=DAEMOT Toolset
  gb1 : BusSelector  OutputSignals=mdot_kgps,T_C,P_kPa
  gp1 : Terminator
  n-D Lookup Table1 : Lookup_n-D  Commented=on  BreakpointsForDimension1=Fluid.P  BreakpointsForDimension2=Fluid.T  BreakpointsForDimension3=[5, 7]  Table=Fluid.C_pt  ExtrapMethod=Clip  UseLastTableValue=on  RndMeth=Simplest  InputSameDT=on
  n-D Lookup Table2 : Lookup_n-D  Commented=on  BreakpointsForDimension1=Fluid.P  BreakpointsForDimension2=Fluid.T  BreakpointsForDimension3=[5, 7]  Table=Fluid.Rho_pt  ExtrapMethod=Clip  UseLastTableValue=on  RndMeth=Simplest  InputSameDT=on
  Out1 : Outport  VectorParamsAs1DForOutWhenUnconnected=off
  wires:
  b1/1 -> Out1/1
  [M_out1] -> b1/1  "mdot_kgps"
  gb1/2 -> [T_in1]  "<T_C>"
  [T_tank] -> b1/2  "T_C"
  gb1/1 -> [M_in1]  "<mdot_kgps>"
  In1/1 -> gb1/1
  [P_tank] -> b1/3  "P_kPa"
  gb1/3 -> gp1/1  "<P_kPa>"
  [P_tank] -> Sink1/1
  Source1/1 -> [M_out1]
  Tank/1(x_dot) -> Integrate/1
  Integrate/1 -> Demux/1, Tank/1(x)
  Demux/1 -> [T_tank]
  Demux/2 -> [P_tank]
  Tank/3(h) -> [h_tank]
  [T_tank] -> n-D Lookup Table2/2, n-D Lookup Table1/2
  [P_tank] -> n-D Lookup Table2/1, n-D Lookup Table1/1
  n-D Lookup Table1/1 -> Tank/6(Cp)
  Tank/2(M) -> [M_tank]
  n-D Lookup Table2/1 -> Tank/7(Rho)
  [T_amb] -> Tank/5(T_amb)
  Bus Creator2/1 -> data_sink1/1
  [T_tank] -> Bus Creator2/1  "T_tank"
  [P_tank] -> Bus Creator2/2  "P_tank"
  [h_tank] -> Bus Creator2/4  "h_tank"
  [M_tank] -> Bus Creator2/3  "M_tank"
  Mux_In_3/1 -> Selector2/1
  Mux_In_1/1 -> Selector1/1
  Mux_In_2/1 -> Tank/3(Mdot_out)
  [M_in1] -> Mux_In_1/1
  [M_out1] -> Mux_In_2/1
  [T_in1] -> Mux_In_3/1
  Selector1/1 -> Tank/2(Mdot_in)
  Selector2/1 -> Tank/4(T_in)
  Q/1 -> Bus Selector/1
  Bus Selector/1 -> [Q_Load]  "<Q_kW>"
  Bus Selector/2 -> Terminator/1  "<Temp>"

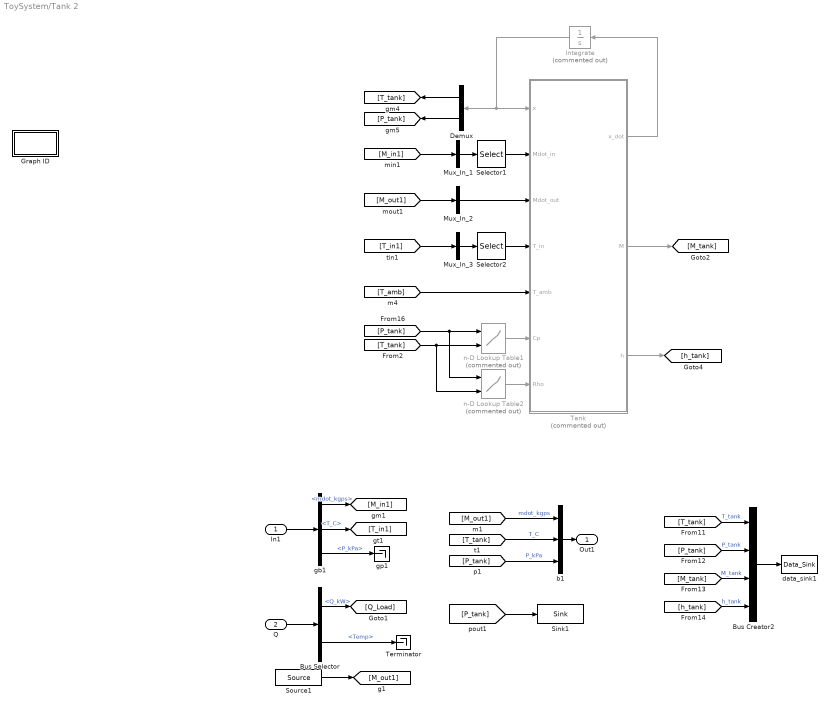
== system ToySystem/Tank 2 ==
  In1 : Inport
  Q : Inport  Port=2
  Bus Creator2 : BusCreator  Inputs=4
  Bus Selector : BusSelector  OutputSignals=Q_kW,Temp
  Demux : Demux  Outputs=2
  Graph ID : Subsystem  mask(Automated Graph Identifier){skip=off, graphType=Tank, downCompType=SplitJunction, downCompPath=ToySystem/Junction, upCompType=SplitJunction,Source, upCompPath=ToySystem/Junction1,ToySystem/Generic Source3, spec=0}
      mask prompts: skip "Skip this block?"; graphType "Graph Type"; downCompType "Downstream Component Type"; downCompPath "Downstream Component Path"; upCompType "Upstream Component Type"; upCompPath "Upstream Component Path"; spec "Special"
      mask help: This block is used to generate directed graphs from DAEMOT models.
      mask init:
      | graph_connections()
      mask TypeOptions graphType: Tank | HeatExchanger | HeatLoad | SplitJunction | Source | Sink
      mask Callback graphType:
      | % grab the Simulink Mask object for this block
      | maskObj = Simulink.Mask.get(gcb);
      | 
      | % assign the popup with a list of graph options
      | maskObj.Parameters(2).TypeOptions = generateGraphList();
  Integrate : Integrator  Commented=on  InitialCondition=[T_init P_init]
  Mux_In_1 : Mux  Inputs=1
  Mux_In_2 : Mux  Inputs=1
  Mux_In_3 : Mux  Inputs=1
  Selector1 : Selector  InputPortWidth=1  IndexOptions=Index vector (dialog)  Indices=[1 ]  OutputSizes=1
  Selector2 : Selector  InputPortWidth=1  IndexOptions=Index vector (dialog)  Indices=[1 ]  OutputSizes=1
  Sink1 : DAEMOT_Lib/Support Functions/Sink
      settings: SourceProductName=DAEMOT Toolset
  Source1 : DAEMOT_Lib/Support Functions/Source
      settings: SourceProductName=DAEMOT Toolset
  Tank : MATLAB Function  Commented=on  TreatAsAtomicUnit=on
  Terminator : Terminator
  b1 : BusCreator  Inputs=3
  data_sink1 : DAEMOT_Lib/Support Functions/Data_Sink
      settings: SourceProductName=DAEMOT Toolset
  gb1 : BusSelector  OutputSignals=mdot_kgps,T_C,P_kPa
  gp1 : Terminator
  n-D Lookup Table1 : Lookup_n-D  Commented=on  BreakpointsForDimension1=Fluid.P  BreakpointsForDimension2=Fluid.T  BreakpointsForDimension3=[5, 7]  Table=Fluid.C_pt  ExtrapMethod=Clip  UseLastTableValue=on  RndMeth=Simplest  InputSameDT=on
  n-D Lookup Table2 : Lookup_n-D  Commented=on  BreakpointsForDimension1=Fluid.P  BreakpointsForDimension2=Fluid.T  BreakpointsForDimension3=[5, 7]  Table=Fluid.Rho_pt  ExtrapMethod=Clip  UseLastTableValue=on  RndMeth=Simplest  InputSameDT=on
  Out1 : Outport  VectorParamsAs1DForOutWhenUnconnected=off
  wires:
  Bus Selector/2 -> Terminator/1  "<Temp>"
  Bus Selector/1 -> [Q_Load]  "<Q_kW>"
  Q/1 -> Bus Selector/1
  Selector2/1 -> Tank/4(T_in)
  Selector1/1 -> Tank/2(Mdot_in)
  [T_in1] -> Mux_In_3/1
  [M_out1] -> Mux_In_2/1
  [M_in1] -> Mux_In_1/1
  Mux_In_2/1 -> Tank/3(Mdot_out)
  Mux_In_1/1 -> Selector1/1
  Mux_In_3/1 -> Selector2/1
  [M_tank] -> Bus Creator2/3  "M_tank"
  [h_tank] -> Bus Creator2/4  "h_tank"
  [P_tank] -> Bus Creator2/2  "P_tank"
  [T_tank] -> Bus Creator2/1  "T_tank"
  Bus Creator2/1 -> data_sink1/1
  [T_amb] -> Tank/5(T_amb)
  n-D Lookup Table2/1 -> Tank/7(Rho)
  Tank/2(M) -> [M_tank]
  n-D Lookup Table1/1 -> Tank/6(Cp)
  [P_tank] -> n-D Lookup Table1/1, n-D Lookup Table2/1
  [T_tank] -> n-D Lookup Table1/2, n-D Lookup Table2/2
  Tank/3(h) -> [h_tank]
  Demux/2 -> [P_tank]
  Demux/1 -> [T_tank]
  Integrate/1 -> Tank/1(x), Demux/1
  Tank/1(x_dot) -> Integrate/1
  Source1/1 -> [M_out1]
  [P_tank] -> Sink1/1
  gb1/3 -> gp1/1  "<P_kPa>"
  [P_tank] -> b1/3  "P_kPa"
  In1/1 -> gb1/1
  gb1/1 -> [M_in1]  "<mdot_kgps>"
  [T_tank] -> b1/2  "T_C"
  gb1/2 -> [T_in1]  "<T_C>"
  [M_out1] -> b1/1  "mdot_kgps"
  b1/1 -> Out1/1

== system ToySystem/Cold Plate/Graph ID ==

== system ToySystem/Generic Sink/Graph ID ==

== system ToySystem/Generic Sink/Sink1 ==
  In1 : Inport
  tag scope: gdata_ToySystemGenericSinkSink1=global
  wires:
  In1/1 -> [gdata_ToySystemGenericSinkSink1]

== system ToySystem/Generic Source/Graph ID ==

== system ToySystem/Generic Source/Source1 ==
  Out1 : Outport  VectorParamsAs1DForOutWhenUnconnected=off
  wires:
  [gdata_ToySystemHXSink1] -> Out1/1

== system ToySystem/Generic Source1/Graph ID ==

== system ToySystem/Generic Source1/Source1 ==
  Out1 : Outport  VectorParamsAs1DForOutWhenUnconnected=off
  wires:
  [gdata_ToySystemColdPlateSink2] -> Out1/1

== system ToySystem/Generic Source2/Graph ID ==

== system ToySystem/Generic Source2/Source1 ==
  Out1 : Outport  VectorParamsAs1DForOutWhenUnconnected=off
  wires:
  [gdata_ToySystemColdPlateSink2] -> Out1/1

== system ToySystem/Generic Source3/Graph ID ==

== system ToySystem/Generic Source3/Source1 ==
  Out1 : Outport  VectorParamsAs1DForOutWhenUnconnected=off
  wires:
  [gdata_ToySystemColdPlateSink2] -> Out1/1

== system ToySystem/HX/Graph ID ==

== system ToySystem/Junction/Graph ID ==

== system ToySystem/Junction/Source1 ==
  Out1 : Outport  VectorParamsAs1DForOutWhenUnconnected=off
  wires:
  [gdata_ToySystemHXSink2] -> Out1/1

== system ToySystem/Junction1/Graph ID ==

== system ToySystem/Junction1/Source1 ==
  Out1 : Outport  VectorParamsAs1DForOutWhenUnconnected=off
  wires:
  [gdata_ToySystemTank1Sink1] -> Out1/1

== system ToySystem/Tank 1/Graph ID ==

== system ToySystem/Tank 2/Graph ID ==

== matlab function ToySystem/Tank 2/Tank ==
  data: x input; x_dot output; Mdot_in input; Mdot_out input; T_in input; T_amb input; Cp input; M output; h output; Rho input; H parameter; D parameter; Pamb parameter
function [x_dot,M,h]= Tank(x,Mdot_in,Mdot_out,T_in,T_amb,Cp,Rho,H,D,Pamb)

% Constants and Conversions
Mdot_in_tot     = sum(Mdot_in);     % Total mass flow rate in
Mdot_out_tot    = sum(Mdot_out);    % Total mass flow rate out
A_cross = pi*D^2/4;             % Cross-sectional area
Cp      = 1000*Cp;              % Convert Cp from J/g*K to J/kg*K
g       = 9.81;                 % Gravitational acceleration

% Parse states
T      = x(1);                  % Temperature of the tank
P      = x(2);                  % Pressure at bottom of the tank

% Calculate outputs
h = 1000*(P-Pamb)/(Rho*g);      % Tank height
M = Rho*A_cross*h;              % Tank mass

% Additional intermediate variable calculations
A_ht    = pi*h*D;               % Heat transfer area          

% Calculate state derivatives
T_dot = ((dot(Mdot_in,T_in)-sum(Mdot_in)*T)-H*A_ht*(T-T_amb)/Cp)/M;    % Tank temperature
P_dot  = (Mdot_in_tot-Mdot_out_tot)*g/(1000*A_cross);        % Tank pressure

% Mux state derivatives
x_dot  = [T_dot,P_dot];

end

== matlab function ToySystem/Junction/Dynamic_Flow_Split_Junction ==
  data: x input; Mdot_in input; Mdot_out input; T_in input; x_dot output; D parameter; L parameter; t parameter; E parameter; v parameter; rho input; E_fluid input
function x_dot  = Dynamic_Flow_Split_Junction(x,Mdot_in,Mdot_out,T_in,D,L,t,E,v,rho,E_fluid)

% Constants and Conversions
Mdot_in_tot     = sum(Mdot_in);     % Total mass flow rate in
Mdot_out_tot    = sum(Mdot_out);    % Total mass flow rate out
V               = pi*D^2/4*L;       % Volume

% Parse states
T      = x(1);                  % Temperature of the tank
P      = x(2);                  % Pressure at bottom of the tank

% Calculate state derivatives
T_dot = (dot(Mdot_in,T_in)-sum(Mdot_out)*T)/(rho*V);  % Split/Junc temperature
P_dot = (Mdot_in_tot-Mdot_out_tot)/(V*rho*(1/E_fluid+D*(1-v/2)/(t*E))); % Split/Junc pressure

% Mux state derivatives
x_dot  = [T_dot,P_dot];

end

== matlab function ToySystem/Junction1/Dynamic_Flow_Split_Junction ==
  data: x input; Mdot_in input; Mdot_out input; T_in input; x_dot output; D parameter; L parameter; t parameter; E parameter; v parameter; rho input; E_fluid input
function x_dot  = Dynamic_Flow_Split_Junction(x,Mdot_in,Mdot_out,T_in,D,L,t,E,v,rho,E_fluid)

% Constants and Conversions
Mdot_in_tot     = sum(Mdot_in);     % Total mass flow rate in
Mdot_out_tot    = sum(Mdot_out);    % Total mass flow rate out
V               = pi*D^2/4*L;       % Volume

% Parse states
T      = x(1);                  % Temperature of the tank
P      = x(2);                  % Pressure at bottom of the tank

% Calculate state derivatives
T_dot = (dot(Mdot_in,T_in)-sum(Mdot_out)*T)/(rho*V);  % Split/Junc temperature
P_dot = (Mdot_in_tot-Mdot_out_tot)/(V*rho*(1/E_fluid+D*(1-v/2)/(t*E))); % Split/Junc pressure

% Mux state derivatives
x_dot  = [T_dot,P_dot];

end

== matlab function ToySystem/HX/HX ==
  data: x input; x_dot output; P_in input size=2; Mdot_down input size=2; Mdot input; T_in input size=2; H output; mu input size=2; k input size=2; Cp input size=2; Rho input size=2; E_fluid input size=2; M_wall parameter; Cp_wall parameter; Pass1 parameter; Pass2 parameter; f1 parameter; f2 parameter; KL1 parameter; KL2 parameter; b1 parameter; b2 parameter; W1 parameter; W2 parameter; L1 parameter; L2 parameter; Nu_lam1 parameter; Nu_lam2 parameter; dH1 parameter; dH2 parameter; HTC_method1 parameter; HTC_method2 parameter; HTC1 parameter; HTC2 parameter
function [x_dot,H]  = HX(x,P_in,Mdot_down,Mdot,T_in,mu,k,Cp,Rho,E_fluid,M_wall,Cp_wall,Pass1,Pass2,f1,f2,KL1,KL2,b1,b2,W1,W2,L1,L2,Nu_lam1,Nu_lam2,dH1,dH2,HTC_method1, HTC_method2, HTC1, HTC2)

% Parse data
P_in1       = P_in(1);
P_in2       = P_in(2);
Mdot_down1  = Mdot_down(1);
Mdot_down2  = Mdot_down(2);
Mdot1       = Mdot(1);
Mdot2       = Mdot(2);
T_in1       = T_in(1);
T_in2       = T_in(2);
mu1         = mu(1);
mu2         = mu(2);
k1          = k(1);
k2          = k(2);
Cp1         = Cp(1);
Cp2         = Cp(2);
Rho1        = Rho(1);
Rho2        = Rho(2);
E_fluid1    = E_fluid(1);
E_fluid2    = E_fluid(2);

% Constants and Conversions
Mdot_down1_pass = Mdot_down1/Pass1;
Mdot_down2_pass = Mdot_down2/Pass2;
Mdot1_pass = Mdot1/Pass1;
Mdot2_pass = Mdot2/Pass2;
g        = 9.81;                   % Gravitational acceleration [m/s^2]
A_ht1    = L1*(2*b1+2*W1);         % Heat transfer area
A_ht2    = L2*(2*b2+2*W2);         % Heat transfer area
V1       = L1*b1*W1;               % Volume per pass
V2       = L2*b2*W2;               % Volume per pass
Cp1      = 1000*Cp1;               % Convert Cp from J/g*K to J/kg*K
Cp2      = 1000*Cp2;               % Convert Cp from J/g*K to J/kg*K
k1       = 1000*k1;                % Convert k from kW/m*K to W/m*K
k2       = 1000*k2;                % Convert k from kW/m*K to W/m*K
C_wall   = M_wall*Cp_wall;         % Heat Capacitance (kJ/K)
C_wall   = 1000*C_wall;            % Covnert heat capacitance from kJ/K to J/K
D1       = 4*b1*W1/(2*b1+2*W1);    % Hydraulic diameter (side 1) (see Incropera, Eq. 8.66)
D2       = 4*b2*W2/(2*b2+2*W2);    % Hydraulic diameter (side 2) (see Incropera, Eq. 8.66)

% Parse states
Tw      = x(1);                 % Wall temperature
P1      = x(2);                 % Outlet pressure (side 1)
P2      = x(3);                 % Outlet pressure (side 2)
T1      = x(4);                 % Outlet temperature (side 1)
T2      = x(5);                 % Outlet temperature (side 2)

% Additional intermediate variable calculations
dP1         = (P_in1-P1)*1000;      % Pressure differential (side 1) [Pa]
dP2         = (P_in2-P2)*1000;      % Pressure differential (side 2) [Pa]
dP1         = dP1 + Rho1*g*dH1;     % Pressure differential corrected for hieght
dP2         = dP2 + Rho2*g*dH2;     % Pressure differential corrected for hieght
um1         = sign(dP1)*sqrt_Lip(2*abs(dP1)/(Rho1*(f1*L1/D1+KL1)));   % Fluid velocity (side 1) [m/s]
um2         = sign(dP2)*sqrt_Lip(2*abs(dP2)/(Rho2*(f2*L2/D2+KL2)));   % Fluid velocity (side 2) [m/s]
Re1         = Rho1*abs(um1)*D1/mu1;      % Reynolds number (side 1)
Re2         = Rho2*abs(um2)*D2/mu2;      % Reynolds number (side 1)
Pr1         = Cp1*mu1/k1;           % Prandtl number (side 1) (see Incropera, Table 6.2)
Pr2         = Cp2*mu2/k2;           % Prandtl number (side 2) (see Incropera, Table 6.2)

% Gneilinski
if Re1 < 2300
    Nu1 = Nu_lam1; % (inteprolated from Incropera, Table 8.1 in initialization)
else
    Nu1 = (f1/8)*(Re1-1000)*Pr1 / (1+12.7*(f1/8)^.5*(Pr1^(2/3)-1)); % (see Incropera, Eq. 8.62)
end
if Re2 < 2300
    Nu2 = Nu_lam2; % (inteprolated from Incropera, Table 8.1 in initialization)
else
    Nu2 = (f2/8)*(Re2-1000)*Pr2 / (1+12.7*(f2/8)^.5*(Pr2^(2/3)-1)); % (see Incropera, Eq. 8.62)
end

% Longo Correlation
% Nu1 = 0.277*Re1^0.766*Pr1^0.333;
% Nu2 = 0.277*Re2^0.766*Pr2^0.333;

% % Manglik Correlation
% Nu1 = 0.44*Re1^0.5*Pr1^0.333;
% Nu2 = 0.44*Re2^0.5*Pr2^0.333;

% Calculate outputs
if HTC_method1 == 0
    H1      = Nu1*k1/D1;        % Heat transfer coefficient (see Incropera, Table 6.2)
else
    H1 = HTC1;
end
if HTC_method2 == 0
    H2      = Nu2*k2/D2;        % Heat transfer coefficient (see Incropera, Table 6.2)
else
    H2 = HTC2;
end
H       = [H1 H2];

% Calculate state derivatives
Tw_dot = ( H1*A_ht1*(T1-Tw) + H2*A_ht2*(T2-Tw) )/C_wall;    % Wall temperature
P1_dot = (Mdot1_pass-Mdot_down1_pass)/(V1*Rho1/E_fluid1);   % Outlet pressure (side 1)
P2_dot = (Mdot2_pass-Mdot_down2_pass)/(V2*Rho2/E_fluid2);   % Outlet pressure (side 2)
Tout1_dot = (Mdot1_pass*(T_in1-T1)+H1*A_ht1/Cp1*(Tw-T1))/(V1*Rho1);   % Outlet temperature (side 1)
Tout2_dot = (Mdot2_pass*(T_in2-T2)+H2*A_ht2/Cp2*(Tw-T2))/(V2*Rho2);   % Outlet temperature (side 2)

% Mux state derivatives
x_dot  = [Tw_dot,P1_dot,P2_dot,Tout1_dot,Tout2_dot];

end

== matlab function ToySystem/HX/Mdot ==
  data: P_in1 input; P_in2 input; Mdot1_tot output; P_out1 input; P_out2 input; Rho1 input; Rho2 input; f1 parameter; f2 parameter; b1 parameter; b2 parameter; W1 parameter; W2 parameter; L1 parameter; L2 parameter; KL1 parameter; KL2 parameter; Mdot2_tot output; Pass1 parameter; Pass2 parameter; dH1 parameter; dH2 parameter
function [Mdot1_tot,Mdot2_tot]   = Mdot(P_in1,P_in2,P_out1,P_out2,Rho1,Rho2,f1,f2,b1,b2,W1,W2,L1,L2,KL1,KL2,Pass1,Pass2,dH1,dH2)

% Constants and Conversions
g           = 9.81;                 % Gravitational acceleration [m/s^2]
D1 = 4*b1*W1/(2*b1+2*W1);           % (see Incropera, Eq. 8.66)
D2 = 4*b2*W2/(2*b2+2*W2);           % (see Incropera, Eq. 8.66)
dP1         = (P_in1-P_out1)*1000;  % Pressure differential (side 1) [Pa]
dP2         = (P_in2-P_out2)*1000;  % Pressure differential (side 2) [Pa]
dP1         = dP1 + Rho1*g*dH1;     % Pressure differential corrected for hieght
dP2         = dP2 + Rho2*g*dH2;     % Pressure differential corrected for hieght
um1         = max(0,sign(dP1)*sqrt_Lip(2*abs(dP1)/(Rho1*(f1*L1/D1+KL1)))); % Fluid velocity (side 1) [m/s]
um2         = max(0,sign(dP2)*sqrt_Lip(2*abs(dP2)/(Rho2*(f2*L2/D2+KL2)))); % Fluid velocity (side 2) [m/s]
Mdot1_pass  = um1*Rho1*b1*W1;       % Mass flow rate per pass (side 1) [kg/s]
Mdot2_pass  = um2*Rho2*b2*W2;       % Mass flow rate per pass (side 2) [kg/s]

% Calculate outputs
Mdot1_tot = Mdot1_pass*Pass1;       % Total mass flow rate (side 1) [kg/s]
Mdot2_tot = Mdot2_pass*Pass2;       % Total mass flow rate (side 2) [kg/s]

end

== matlab function ToySystem/Tank 1/Tank ==
  data: x input; x_dot output; Mdot_in input; Mdot_out input; T_in input; T_amb input; Cp input; M output; h output; Rho input; H parameter; D parameter; Pamb parameter
function [x_dot,M,h]= Tank(x,Mdot_in,Mdot_out,T_in,T_amb,Cp,Rho,H,D,Pamb)

% Constants and Conversions
Mdot_in_tot     = sum(Mdot_in);     % Total mass flow rate in
Mdot_out_tot    = sum(Mdot_out);    % Total mass flow rate out
A_cross = pi*D^2/4;             % Cross-sectional area
Cp      = 1000*Cp;              % Convert Cp from J/g*K to J/kg*K
g       = 9.81;                 % Gravitational acceleration

% Parse states
T      = x(1);                  % Temperature of the tank
P      = x(2);                  % Pressure at bottom of the tank

% Calculate outputs
h = 1000*(P-Pamb)/(Rho*g);      % Tank height
M = Rho*A_cross*h;              % Tank mass

% Additional intermediate variable calculations
A_ht    = pi*h*D;               % Heat transfer area          

% Calculate state derivatives
T_dot = ((dot(Mdot_in,T_in)-sum(Mdot_in)*T)-H*A_ht*(T-T_amb)/Cp)/M;    % Tank temperature
P_dot  = (Mdot_in_tot-Mdot_out_tot)*g/(1000*A_cross);        % Tank pressure

% Mux state derivatives
x_dot  = [T_dot,P_dot];

end

== matlab function ToySystem/Cold Plate/Cold_Plate ==
  data: x input; Q_load input; x_dot output; P_in input; Mdot_down input; Mdot input; T_in input; H output; mu input; k input; Cp input; Rho input; E_fluid input; f parameter; M_wall parameter; Cp_wall parameter; D parameter; L parameter; t parameter; E parameter; v parameter; KL parameter; dH parameter; PAF parameter; Re output; HTC_method parameter; HTC parameter
function [x_dot,H,Re]  = Cold_Plate(x,Q_load,P_in,Mdot_down,Mdot,T_in,mu,k,Cp,Rho,E_fluid,f,M_wall,Cp_wall,D,L,t,E,v,KL,dH,PAF,HTC_method, HTC)

% Constants and Conversions
g       = 9.81;                 % Gravitational acceleration [m/s^2]
A_ht    = pi*L*D;                  % Heat transfer area
V       = L*pi*D^2/4;              % Volume
C_wall  = M_wall*Cp_wall;          % Heat Capacitance (kJ/K)
C_wall  = 1000*C_wall;             % Covnert heat capacitance from kJ/K to J/K
Q_load  = 1000*Q_load;             % Convert load from kW to W
Cp      = 1000*Cp;                 % Convert Cp from J/g*K to J/kg*K
k       = 1000*k;                  % Convert k from kW/m*K to W/m*K

% Parse states
T       = x(1);                 % Temperature of the tank
P       = x(2);                 % Pressure at bottom of the tank
Tw      = x(3);                 % Wall temperature

% Additional intermediate variable calculations
dP      = (P_in-P)*1000;        % Pressure difference [Pa]
dP      = dP + Rho*g*dH;        % Pressure differential corrected for hieght
um      = sign(dP)*sqrt_Lip(2*abs(dP)/(Rho*(f*L/D+KL)));    % Fluid velocity [m/s]
Re      = Rho*um*D/mu;          % Reynolds number
Pr      = Cp*mu/k;              % Prandtl number (see Incropera, Table 6.2)

if HTC_method == 0
    if Re < 2300
        Nu = 3.66; % (see Incropera, Eq. 8.55)
    else
        Nu = (f/8)*(Re-1000)*Pr / (1+12.7*(f/8)^.5*(Pr^(2/3)-1)); % (see Incropera, Eq. 8.62)  
    end
    H  = PAF*Nu*k/D;            % Heat transfer coefficient (see Incropera, Table 6.2)
else
    H = HTC; 
    % modified by JK 11/11/17
    % H = HTC*Mdot;
end

% Calculate state derivatives
T_dot   = (Mdot*(T_in-T)+H*A_ht/Cp*(Tw-T))/(V*Rho);     % Outlet temperature 
P_dot   = (Mdot-Mdot_down)/(V*Rho*(1/E_fluid+D*(1-v/2)/(t*E))); % Outlet pressure
Tw_dot  = (Q_load - H*A_ht*(Tw-T))/C_wall;              % Wall temperature

% Mux state derivatives
x_dot  = [T_dot,P_dot,Tw_dot];

end

== matlab function ToySystem/Cold Plate/Mdot ==
  data: P_in input; P_out input; Mdot output; Rho input; f parameter; D parameter; L parameter; KL parameter; dH parameter
function Mdot = Mdot(P_in,P_out,Rho,f,D,L,KL,dH)

% Constants and Conversions
g           = 9.81;                 % Gravitational acceleration [m/s^2]
A_cross     = pi*D^2/4;             % Cross sectional area
dP          = (P_in-P_out)*1000;    % Pressure differential [Pa]
dP          = dP + Rho*g*dH;        % Pressure differential corrected for hieght
um          = max(0,sign(dP)*sqrt_Lip(2*abs(dP)/(Rho*(f*L/D+KL))));    % Fluid velocity [m/s]

% Calculate outputs
Mdot        = um*Rho*A_cross;       % Mass flow rate [kg/s]

end
